simulink model "Receiver_UnderTest_Fixed"  (R2019b)
settings: Solver=FixedStepDiscrete  StartTime=0.0  StopTime=0.056285  RelTol=1e-3
InitFcn:
  | modelSettings
undefined symbols (not defined in the file): RadioSampleRate
libraries: commsource2 x1, RxTxFixedPointLibrary_noscopes x1
settings Model: DataTypeOverride=Off  MinMaxOverflowLogging=MinMaxAndOverflow  FPTRunName=NoOverride  Creator=tcollins  LastModifiedBy=bhisma
settings DataIOCC: SaveFormat=Array  SaveOutput=off  SaveTime=off  ReturnWorkspaceOutputs=off
settings OptimizationCC: BlockReduction=off  ConditionallyExecuteInputs=off  DefaultParameterBehavior=Inlined
settings DebuggingCC: AlgebraicLoopMsg=error  SingleTaskRateTransMsg=error  ArithmeticOperatorsInVariantConditions=warning
settings HardwareCC: ProdBitPerPointer=32  ProdBitPerSizeT=32  ProdBitPerPtrDiffT=32  ProdLargestAtomicFloat=None  ProdIntDivRoundTo=Undefined  ProdEndianess=Unspecified  ProdWordSize=32  ProdHWDeviceType=ASIC/FPGA->ASIC/FPGA  ProdEqTarget=off
settings SFSimCC: SimUseLocalCustomCode=off  CustomCodeUndefinedFunction=UseInterfaceOnly
settings RTWCC: RTWUseLocalCustomCode=off
settings CodeAppCC: StateflowObjectComments=on
settings SimscapeCC: SimscapeNormalizeSystem=off

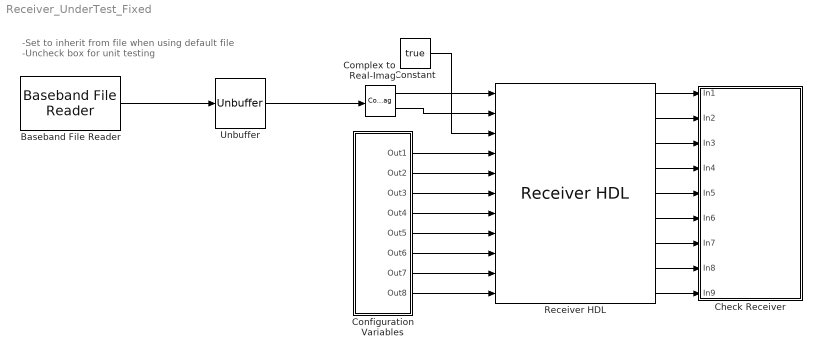
== system Receiver_UnderTest_Fixed ==
  note: -Set to inherit from file when using default file
      | -Uncheck box for unit testing
  Baseband File Reader : commsource2/Baseband File Reader  Filename=PlutoCaptureQPSK.bb  InheritSampleTimeFromFile=off  SampleTime=100000/RadioSampleRate  SamplesPerFrame=100000  CyclicRepetition=off  FileEndOutputPort=off  SimulateUsing=Interpreted execution
      settings: SourceProductName=Communications Toolbox  SourceProductBaseCode=CM
  Check Receiver : Subsystem
  Complex to Real-Imag : ComplexToRealImag
  Configuration Variables : Subsystem
  Constant : Constant  Value=true  SampleTime=1/RadioSampleRate
  Receiver HDL : RxTxFixedPointLibrary_noscopes/Receiver HDL  SystemSampleTime=-1
  Unbuffer : Unbuffer
  wires:
  Constant/1 -> Receiver HDL/3
  Complex to Real-Imag/2 -> Receiver HDL/2
  Baseband File Reader/1 -> Unbuffer/1
  Unbuffer/1 -> Complex to Real-Imag/1
  Configuration Variables/1(Out1) -> Receiver HDL/4
  Configuration Variables/2(Out2) -> Receiver HDL/5
  Configuration Variables/3(Out3) -> Receiver HDL/6
  Complex to Real-Imag/1 -> Receiver HDL/1
  Receiver HDL/1 -> Check Receiver/1(In1)
  Receiver HDL/2 -> Check Receiver/2(In2)
  Receiver HDL/3 -> Check Receiver/3(In3)
  Receiver HDL/5 -> Check Receiver/5(In5)
  Receiver HDL/6 -> Check Receiver/6(In6)
  Configuration Variables/4(Out4) -> Receiver HDL/7
  Configuration Variables/5(Out5) -> Receiver HDL/8
  Receiver HDL/4 -> Check Receiver/4(In4)
  Receiver HDL/7 -> Check Receiver/7(In7)
  Receiver HDL/8 -> Check Receiver/8(In8)
  Receiver HDL/9 -> Check Receiver/9(In9)
  Configuration Variables/6(Out6) -> Receiver HDL/9
  Configuration Variables/7(Out7) -> Receiver HDL/10
  Configuration Variables/8(Out8) -> Receiver HDL/11

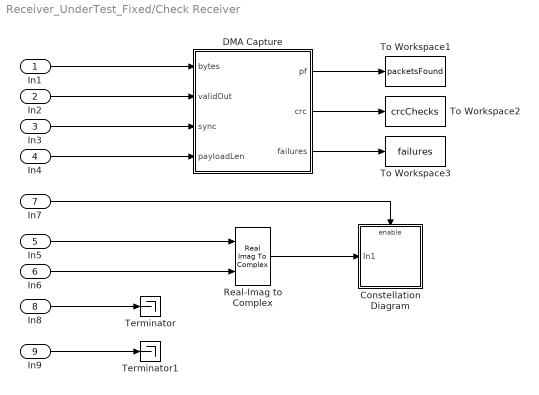
== system Receiver_UnderTest_Fixed/Check Receiver ==
  In1 : Inport
  In2 : Inport  Port=2
  In3 : Inport  Port=3
  In4 : Inport  Port=4
  In5 : Inport  Port=5
  In6 : Inport  Port=6
  In7 : Inport  Port=7
  In8 : Inport  Port=8
  In9 : Inport  Port=9
  Constellation Diagram : Subsystem
  DMA Capture : MATLAB Function  TreatAsAtomicUnit=on
  Real-Imag to Complex : RealImagToComplex
  Terminator : Terminator
  Terminator1 : Terminator
  To Workspace1 : ToWorkspace  VariableName=packetsFound  SaveFormat=Timeseries  SampleTime=-1
  To Workspace2 : ToWorkspace  VariableName=crcChecks  SaveFormat=Timeseries  SampleTime=-1
  To Workspace3 : ToWorkspace  VariableName=failures  SaveFormat=Timeseries  SampleTime=-1
  wires:
  Real-Imag to Complex/1 -> Constellation Diagram/1(In1)
  In5/1 -> Real-Imag to Complex/1
  In3/1 -> DMA Capture/3(sync)
  In7/1 -> Constellation Diagram/Enable
  In2/1 -> DMA Capture/2(validOut)
  In1/1 -> DMA Capture/1(bytes)
  In4/1 -> DMA Capture/4(payloadLen)
  In6/1 -> Real-Imag to Complex/2
  DMA Capture/1(pf) -> To Workspace1/1
  DMA Capture/2(crc) -> To Workspace2/1
  DMA Capture/3(failures) -> To Workspace3/1
  In8/1 -> Terminator/1
  In9/1 -> Terminator1/1

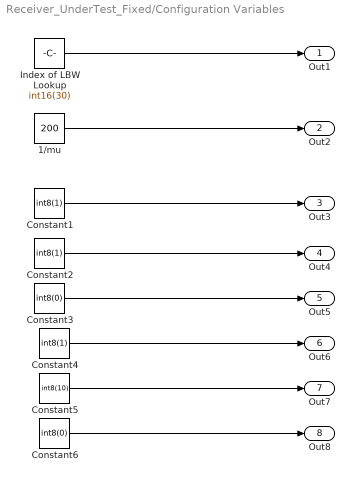
== system Receiver_UnderTest_Fixed/Configuration Variables ==
  1/mu : Constant  Value=200  OutDataTypeStr=int16  SampleTime=-1
  Constant1 : Constant  Value=int8(1)  SampleTime=1/RadioSampleRate
  Constant2 : Constant  Value=int8(1)  SampleTime=1/RadioSampleRate
  Constant3 : Constant  Value=int8(0)  SampleTime=1/RadioSampleRate
  Constant4 : Constant  Value=int8(1)  SampleTime=1/RadioSampleRate
  Constant5 : Constant  Value=int8(10)  SampleTime=1/RadioSampleRate
  Constant6 : Constant  Value=int8(0)  SampleTime=1/RadioSampleRate
  Index of LBW Lookup : Constant  Value=int16(30)  SampleTime=1/RadioSampleRate
  Out1 : Outport  VectorParamsAs1DForOutWhenUnconnected=off
  Out2 : Outport  Port=2  VectorParamsAs1DForOutWhenUnconnected=off
  Out3 : Outport  Port=3  VectorParamsAs1DForOutWhenUnconnected=off
  Out4 : Outport  Port=4  VectorParamsAs1DForOutWhenUnconnected=off
  Out5 : Outport  Port=5  VectorParamsAs1DForOutWhenUnconnected=off
  Out6 : Outport  Port=6  VectorParamsAs1DForOutWhenUnconnected=off
  Out7 : Outport  Port=7  VectorParamsAs1DForOutWhenUnconnected=off
  Out8 : Outport  Port=8  VectorParamsAs1DForOutWhenUnconnected=off
  wires:
  1/mu/1 -> Out2/1
  Index of LBW Lookup/1 -> Out1/1
  Constant1/1 -> Out3/1
  Constant2/1 -> Out4/1
  Constant3/1 -> Out5/1
  Constant4/1 -> Out6/1
  Constant5/1 -> Out7/1
  Constant6/1 -> Out8/1

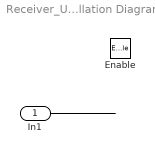
== system Receiver_UnderTest_Fixed/Check Receiver/Constellation Diagram ==
  In1 : Inport
  Enable : EnablePort
  wires:
  In1/1 -> ?

== matlab function Receiver_UnderTest_Fixed/Check Receiver/DMA Capture ==
  data: bytes input; validOut input; sync input; payloadLen input; pf output; crc output; failures output
function [pf, crc, failures] = fcn(bytes, validOut, sync, payloadLen)

persistent frameBuffer byteCounter fullPayloadBits result

bitsInPack = 64;

if isempty(frameBuffer)
    maxFrameBits = (2^16)*8;
    frameBuffer = false(maxFrameBits,1);
    byteCounter = 0;
    fullPayloadBits = uint16(0);
    result = struct('packetsFound',0,...
    'crcChecks',zeros(1,100),'failures',zeros(1,100));
end

if validOut
    if sync
        byteCounter = bitsInPack;
        frameBuffer(1:byteCounter) = bitget(bytes,1:bitsInPack);
        fullPayloadBits = uint16(payloadLen*8);
        
    elseif byteCounter<fullPayloadBits
        frameBuffer(byteCounter+1:byteCounter+bitsInPack) = bitget(bytes,1:bitsInPack);
        byteCounter = byteCounter + bitsInPack;
    else
        result.packetsFound = result.packetsFound + 1;
        if bytes>0
            fprintf('CRC Error (Exterior Check) [Len: %u]\n',fullPayloadBits);
            result.crcChecks(result.packetsFound) = 1;
            result.failures(result.packetsFound) = 4;
        else
            fprintf('Frame passed CRC (Exterior Check) [Len: %u]\n',fullPayloadBits);
        end
    end
end

pf = result.packetsFound;
crc = result.crcChecks;
failures = result.failures;
